simulink model "Synchronism_ETR07"  (R2017b)
settings: Solver=FixedStepAuto  StartTime=0.0  StopTime=10.0  RelTol=1e-3
libraries: simulink x1
settings Model: Creator=cspt  LastModifiedBy=cspt
settings RTWCC: SystemTargetFile=irt.tlc  TemplateMakefile=irt_default_tmf  Description=INTECRIO Real-Time Target
settings STFCustomTargetCC: TargetLangStandard=C99 (ISO)  UtilityFuncGeneration=Shared location  SystemTargetFile=irt.tlc
settings GRTTargetCC: UtilityFuncGeneration=Shared location  ParMdlRefBuildCompliant=off  CompOptLevelCompliant=off  ConcurrentExecutionCompliant=off  CombineOutputUpdateFcns=off  MatFileLogging=off  CPPClassGenCompliant=off  GRTInterface=on  UseToolchainInfoCompliant=off  GenerateASAP2=on

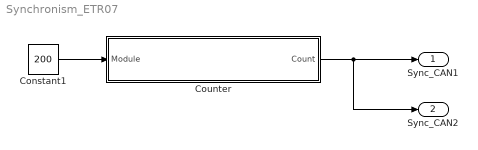
== system Synchronism_ETR07 ==
  Constant1 : Constant  Value=200
  Counter : Subsystem
  Sync_CAN1 : Outport
  Sync_CAN2 : Outport  Port=2
  wires:
  Counter/1(Count) -> Sync_CAN2/1, Sync_CAN1/1
  Constant1/1 -> Counter/1(Module)

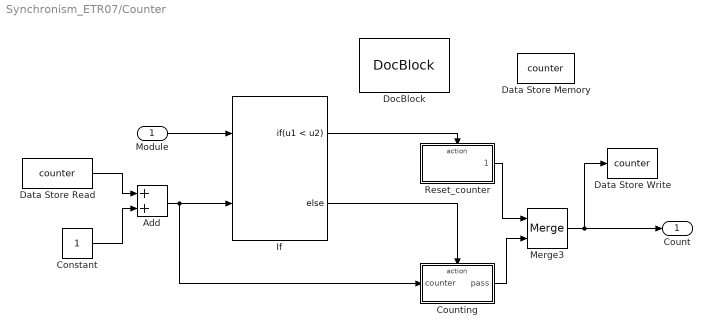
== system Synchronism_ETR07/Counter ==
  Module : Inport
  Add : Sum
  Constant : Constant
  Counting : Subsystem  TreatAsAtomicUnit=on
  Data Store Memory : DataStoreMemory  DataStoreName=counter  ReadBeforeWriteMsg=warning  WriteAfterWriteMsg=warning  WriteAfterReadMsg=warning  ShowAdditionalParam=off
  Data Store Read : DataStoreRead  DataStoreName=counter
  Data Store Write : DataStoreWrite  DataStoreName=counter
  DocBlock : simulink/Model-Wide Utilities/DocBlock  DocumentType=Text
      content=|
      | Per generar la rampa es defineix un contador amb la variable counter
      |
      | Cada vegada que s'executa el model s'agafa el contador i es suma 1.
      | Si aquest valor és més gran que el mòdul del contador vol dir que hem de continuar contant,
      | sinó s'ha de resetejar el contador i posar-lo a 1.
  If : If  NumInputs=2  IfExpression=u1 < u2
  Merge3 : Merge
  Reset_counter : Subsystem  TreatAsAtomicUnit=on
  Count : Outport
  wires:
  Data Store Read/1 -> Add/1
  Constant/1 -> Add/2
  If/1 -> Reset_counter/Action
  If/2 -> Counting/Action
  Reset_counter/1(1) -> Merge3/1
  Counting/1(pass) -> Merge3/2
  Merge3/1 -> Data Store Write/1, Count/1
  Module/1 -> If/1
  Add/1 -> Counting/1(counter), If/2

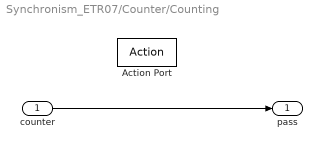
== system Synchronism_ETR07/Counter/Counting ==
  counter : Inport
  Action Port : ActionPort  ActionType=else
  pass : Outport
  wires:
  counter/1 -> pass/1

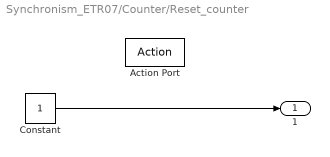
== system Synchronism_ETR07/Counter/Reset_counter ==
  Action Port : ActionPort  ActionType=then
  Constant : Constant
  1 : Outport
  wires:
  Constant/1 -> 1/1
